simulink model "Quadcopter_Plant_x"  (R2022b)
settings: Solver=FixedStepAuto  StartTime=0.0  StopTime=60  FixedStep=.01  RelTol=1e-3
undefined symbols (not defined in the file): CdProp, Cdx, Cdy, Cdz, Ct, DiscIntNeverNeededParam, Earth, Ixx, Iyy, Izz, Jr, larm, mass, WGS84
libraries: sharedtransform x2, aerolibtransform2 x1
settings Model: Creator=aaron  LastModifiedBy=aaron
settings DataIOCC: SaveOutput=off  SaveTime=off
settings DebuggingCC: ModelReferenceExtraNoncontSigs=none

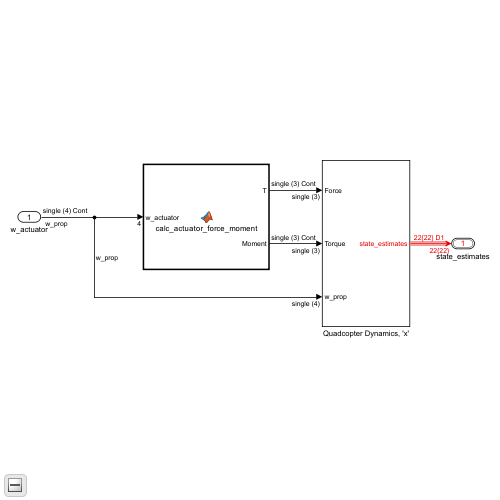
[thumbnail: Simulink's stored preview of the top-level diagram]
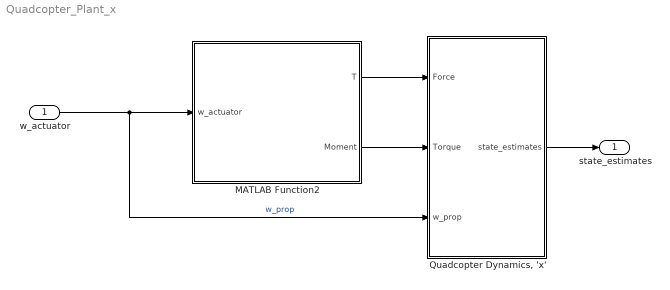
== system Quadcopter_Plant_x ==
  w_actuator : Inport  OutDataTypeStr=single  PortDimensions=4  SampleTime=[0.01,0]
  MATLAB Function2 : MATLAB Function  TreatAsAtomicUnit=on
  "Quadcopter Dynamics, 'x'" : Subsystem
  state_estimates : Outport  OutDataTypeStr=Bus: state_estimates  LockScale=on
  wires:
  MATLAB Function2/1(T) -> "Quadcopter Dynamics, 'x'"/1(Force)
  MATLAB Function2/2(Moment) -> "Quadcopter Dynamics, 'x'"/2(Torque)
  w_actuator/1 -> "Quadcopter Dynamics, 'x'"/3(w_prop), MATLAB Function2/1(w_actuator)  "w_prop"
  "Quadcopter Dynamics, 'x'"/1(state_estimates) -> state_estimates/1

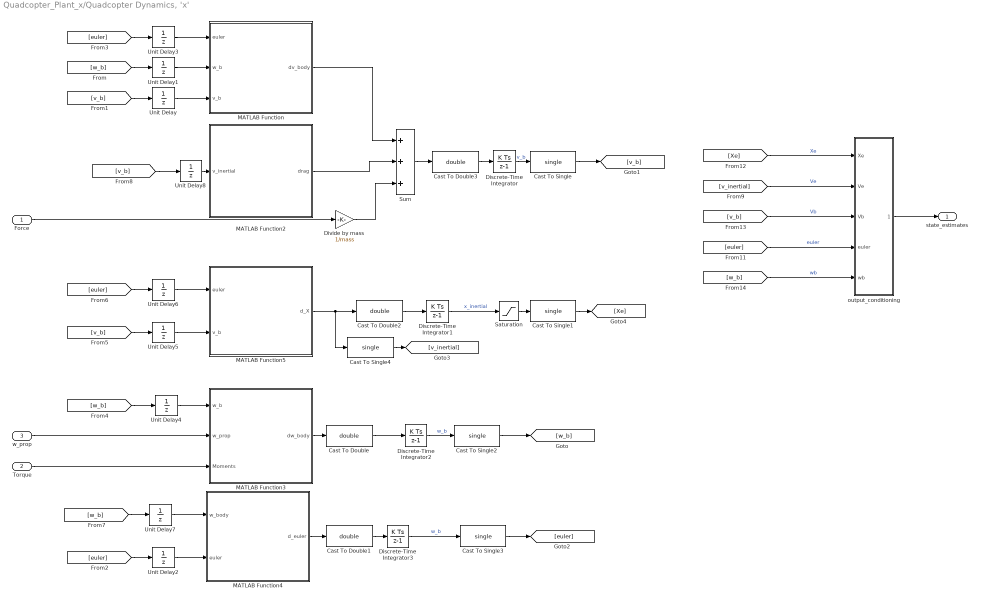
== system Quadcopter_Plant_x/Quadcopter Dynamics, 'x' ==
  Force : Inport  OutDataTypeStr=single
  Torque : Inport  Port=2  OutDataTypeStr=single
  w_prop : Inport  Port=3  OutDataTypeStr=single
  Cast To Double{,1..3} (4 alike) : DataTypeConversion  OutDataTypeStr=double  SaturateOnIntegerOverflow=off  RndMeth=Floor
  Cast To Single{,1..4} (5 alike) : DataTypeConversion  OutDataTypeStr=single  SaturateOnIntegerOverflow=off  RndMeth=Floor
  Discrete-Time Integrator : DiscreteIntegrator  SampleTime=.01  OutDataTypeStr=single  ICPrevOutput=DiscIntNeverNeededParam  ICPrevScaledInput=DiscIntNeverNeededParam
  Discrete-Time Integrator1 : DiscreteIntegrator  SampleTime=.01  OutDataTypeStr=single  LimitOutput=on  UpperSaturationLimit=[inf inf 0]  LowerSaturationLimit=[-inf -inf -inf]  ICPrevOutput=DiscIntNeverNeededParam  ICPrevScaledInput=DiscIntNeverNeededParam
  Discrete-Time Integrator2 : DiscreteIntegrator  SampleTime=.01  OutDataTypeStr=single  ICPrevOutput=DiscIntNeverNeededParam  ICPrevScaledInput=DiscIntNeverNeededParam
  Discrete-Time Integrator3 : DiscreteIntegrator  SampleTime=.01  OutDataTypeStr=single  ICPrevOutput=DiscIntNeverNeededParam  ICPrevScaledInput=DiscIntNeverNeededParam
  Divide by mass : Gain  Gain=1/mass  OutDataTypeStr=single
  MATLAB Function : MATLAB Function  TreatAsAtomicUnit=on
  MATLAB Function2 : MATLAB Function  TreatAsAtomicUnit=on
  MATLAB Function3 : MATLAB Function  TreatAsAtomicUnit=on
  MATLAB Function4 : MATLAB Function  TreatAsAtomicUnit=on
  MATLAB Function5 : MATLAB Function  TreatAsAtomicUnit=on
  Saturation : Saturate  UpperLimit=[inf inf 0]  LowerLimit=-inf
  Sum : Sum  Inputs=+++
  Unit Delay{,1..8} (9 alike) : UnitDelay  SampleTime=-1  HasFrameUpgradeWarning=on
  output_conditioning : Subsystem
  state_estimates : Outport  OutDataTypeStr=Bus: state_estimates  LockScale=on
  wires:
  Divide by mass/1 -> Sum/3
  Torque/1 -> MATLAB Function3/3(Moments)
  MATLAB Function3/1(dw_body) -> Cast To Double/1
  Discrete-Time Integrator1/1 -> Saturation/1  "x_inertial"
  [v_b] -> Unit Delay8/1
  Unit Delay8/1 -> MATLAB Function2/1(v_inertial)
  MATLAB Function5/1(d_X) -> Cast To Single4/1, Cast To Double2/1
  Unit Delay7/1 -> MATLAB Function4/1(w_body)
  [w_b] -> Unit Delay7/1
  Unit Delay6/1 -> MATLAB Function5/1(euler)
  [euler] -> Unit Delay6/1
  Unit Delay5/1 -> MATLAB Function5/2(v_b)
  [v_b] -> Unit Delay5/1
  Unit Delay4/1 -> MATLAB Function3/1(w_b)
  [w_b] -> Unit Delay4/1
  w_prop/1 -> MATLAB Function3/2(w_prop)
  [euler] -> Unit Delay2/1
  Unit Delay3/1 -> MATLAB Function/1(euler)
  [euler] -> Unit Delay3/1
  Unit Delay2/1 -> MATLAB Function4/2(euler)
  MATLAB Function4/1(d_euler) -> Cast To Double1/1
  [v_b] -> Unit Delay/1
  Discrete-Time Integrator/1 -> Cast To Single/1  "v_b"
  [w_b] -> Unit Delay1/1
  Unit Delay1/1 -> MATLAB Function/2(w_b)
  Discrete-Time Integrator2/1 -> Cast To Single2/1  "w_b"
  Sum/1 -> Cast To Double3/1
  Force/1 -> Divide by mass/1
  Unit Delay/1 -> MATLAB Function/3(v_b)
  MATLAB Function2/1(drag) -> Sum/2
  MATLAB Function/1(dv_body) -> Sum/1
  Saturation/1 -> Cast To Single1/1
  [Xe] -> output_conditioning/1(Xe)  "Xe"
  [v_inertial] -> output_conditioning/2(Ve)  "Ve"
  [v_b] -> output_conditioning/3(Vb)  "Vb"
  [euler] -> output_conditioning/4(euler)  "euler"
  [w_b] -> output_conditioning/5(wb)  "wb"
  output_conditioning/1(state_estimates) -> state_estimates/1
  Cast To Single/1 -> [v_b]
  Cast To Single1/1 -> [Xe]
  Cast To Single2/1 -> [w_b]
  Discrete-Time Integrator3/1 -> Cast To Single3/1  "w_b"
  Cast To Single3/1 -> [euler]
  Cast To Double/1 -> Discrete-Time Integrator2/1
  Cast To Double1/1 -> Discrete-Time Integrator3/1
  Cast To Single4/1 -> [v_inertial]
  Cast To Double2/1 -> Discrete-Time Integrator1/1
  Cast To Double3/1 -> Discrete-Time Integrator/1

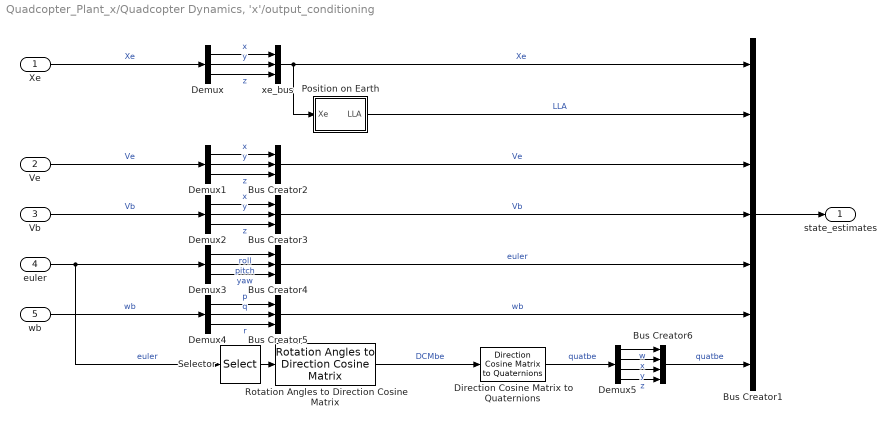
== system Quadcopter_Plant_x/Quadcopter Dynamics, 'x'/output_conditioning ==
  Xe : Inport
  Ve : Inport  Port=2
  Vb : Inport  Port=3
  euler : Inport  Port=4
  wb : Inport  Port=5
  Bus Creator1 : BusCreator  Inputs=7  OutDataTypeStr=Bus: state_estimates
  Bus Creator2 : BusCreator  Inputs=3  OutDataTypeStr=Bus: Velocity
  Bus Creator3 : BusCreator  Inputs=3  OutDataTypeStr=Bus: Velocity
  Bus Creator4 : BusCreator  Inputs=3  OutDataTypeStr=Bus: euler
  Bus Creator5 : BusCreator  Inputs=3  OutDataTypeStr=Bus: body_rates
  Bus Creator6 : BusCreator  Inputs=4  OutDataTypeStr=Bus: quat
  Demux{,1..4} (5 alike) : Demux  Outputs=3
  Demux5 : Demux
  Direction Cosine Matrix to Quaternions : sharedtransform/Direction Cosine Matrix  to Quaternions  aMode=0  action=None  tolerance=eps(2)
      settings: LibrarySourceBlock=|
      | aerolibtransform2/Direction Cosine Matrix
      | to Quaternions
  Position on Earth : Subsystem  Priority=1  TreatAsAtomicUnit=on
  Rotation Angles to Direction Cosine Matrix : sharedtransform/Rotation Angles to Direction Cosine Matrix  rotationOrder=ZYX  aMode=aMode
  Selector : Selector  InputPortWidth=3  IndexOptions=Index vector (dialog)  Indices=[3 2 1]  OutputSizes=1
  xe_bus : BusCreator  Inputs=3  OutDataTypeStr=Bus: Position
  state_estimates : Outport  OutDataTypeStr=Bus: state_estimates  LockScale=on
  wires:
  euler/1 -> Demux3/1, Selector/1  "euler"
  Bus Creator1/1 -> state_estimates/1
  Position on Earth/1(LLA) -> Bus Creator1/2  "LLA"
  Selector/1 -> Rotation Angles to Direction Cosine Matrix/1
  Xe/1 -> Demux/1  "Xe"
  Demux/1 -> xe_bus/1  "x"
  Demux/2 -> xe_bus/2  "y"
  Demux/3 -> xe_bus/3  "z"
  xe_bus/1 -> Bus Creator1/1, Position on Earth/1(Xe)  "Xe"
  Demux1/1 -> Bus Creator2/1  "x"
  Demux1/2 -> Bus Creator2/2  "y"
  Demux1/3 -> Bus Creator2/3  "z"
  Ve/1 -> Demux1/1  "Ve"
  Bus Creator2/1 -> Bus Creator1/3  "Ve"
  Demux2/3 -> Bus Creator3/3  "z"
  Demux2/2 -> Bus Creator3/2  "y"
  Demux2/1 -> Bus Creator3/1  "x"
  Bus Creator3/1 -> Bus Creator1/4  "Vb"
  Vb/1 -> Demux2/1  "Vb"
  Demux3/1 -> Bus Creator4/1  "roll"
  Demux3/2 -> Bus Creator4/2  "pitch"
  Demux3/3 -> Bus Creator4/3  "yaw"
  Bus Creator4/1 -> Bus Creator1/5  "euler"
  wb/1 -> Demux4/1  "wb"
  Bus Creator5/1 -> Bus Creator1/6  "wb"
  Demux4/1 -> Bus Creator5/1  "p"
  Demux4/2 -> Bus Creator5/2  "q"
  Demux4/3 -> Bus Creator5/3  "r"
  Rotation Angles to Direction Cosine Matrix/1 -> Direction Cosine Matrix to Quaternions/1  "DCMbe"
  Demux5/1 -> Bus Creator6/1  "w"
  Demux5/2 -> Bus Creator6/2  "x"
  Demux5/3 -> Bus Creator6/3  "y"
  Demux5/4 -> Bus Creator6/4  "z"
  Bus Creator6/1 -> Bus Creator1/7  "quatbe"
  Direction Cosine Matrix to Quaternions/1 -> Demux5/1  "quatbe"

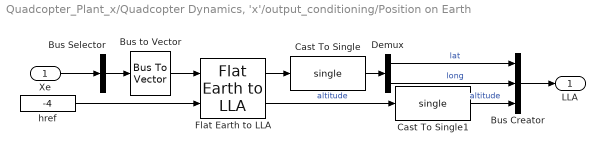
== system Quadcopter_Plant_x/Quadcopter Dynamics, 'x'/output_conditioning/Position on Earth ==
  Xe : Inport  OutDataTypeStr=Bus: Position  Unit=m
  Bus Creator : BusCreator  Inputs=3  OutDataTypeStr=Bus: LLA
  Bus Selector : BusSelector  OutputSignals=x,y,z  OutputAsBus=on
  Bus to Vector : BusToVector
  Cast To Single : DataTypeConversion  OutDataTypeStr=single  SaturateOnIntegerOverflow=off  RndMeth=Floor
  Cast To Single1 : DataTypeConversion  OutDataTypeStr=single  SaturateOnIntegerOverflow=off  RndMeth=Floor
  Demux : Demux  Outputs=2
  Flat Earth to LLA : aerolibtransform2/Flat Earth to LLA  units=Metric (MKS)  ptype=Earth (WGS84)  F=1/298.257223563  R=6378137  refPosPort=off  LL0=[-122.389977, 37.615223]  psi=0
  href : Constant  Value=-4
  LLA : Outport  OutDataTypeStr=Bus: LLA  VectorParamsAs1DForOutWhenUnconnected=off
  wires:
  Bus Creator/1 -> LLA/1
  href/1 -> Flat Earth to LLA/2
  Demux/2 -> Bus Creator/2  "long"
  Flat Earth to LLA/1 -> Cast To Single/1
  Demux/1 -> Bus Creator/1  "lat"
  Flat Earth to LLA/2 -> Cast To Single1/1  "altitude"
  Xe/1 -> Bus Selector/1
  Bus Selector/1 -> Bus to Vector/1
  Bus to Vector/1 -> Flat Earth to LLA/1
  Cast To Single/1 -> Demux/1
  Cast To Single1/1 -> Bus Creator/3  "altitude"

== matlab function Quadcopter_Plant_x/MATLAB Function2 ==
  data: w_actuator input single; T output single size=3; Moment output single size=3; Ct parameter single; larm parameter single; CdProp parameter single
function [T, Moment] = calc_actuator_force_moment(w_actuator, Ct, larm, CdProp)

K = Ct;
L_arm = larm;
C = CdProp;


w1 = w_actuator(1)^2;
w2 = w_actuator(2)^2;
w3 = w_actuator(3)^2;
w4 = w_actuator(4)^2;

T = [0; 0; -K * (sum(w_actuator.^2))];
L = K*L_arm*(-w1 + w2 + w3 - w4);
M = K*L_arm*(-w1 - w2 + w3 + w4);
N = C*(-w1 - w3 + w2 + w4);

Moment = [L; M; N];

== matlab function Quadcopter_Plant_x/Quadcopter Dynamics, 'x'/MATLAB Function ==
  data: euler input; dv_body output size=3; w_b input; v_b input; g parameter
function dv_body = calc_body_vel_change(euler, w_b, v_b, g)

u = v_b(1);
v = v_b(2);
w = v_b(3);

theta = euler(2);
phi = euler(1);
psi = euler(3);

p = w_b(1);
q = w_b(2);
r = w_b(3);


du = -g*sin(theta)+r*v - q*w;
dv = g*sin(phi)*cos(theta) - r*u + p*w;
dw = g*cos(phi)*cos(theta) + q*u - p*v;

dv_body = [du; dv; dw];

== matlab function Quadcopter_Plant_x/Quadcopter Dynamics, 'x'/MATLAB Function2 ==
  data: v_inertial input single; drag output single size=3; Cdx parameter single; Cdy parameter single; Cdz parameter single; mass parameter single
function drag = calc_drag(v_inertial, Cdx, Cdy, Cdz, mass)

dx = v_inertial(1);
dy = v_inertial(2);
dz = v_inertial(3);

Fd_x = -(1/mass)*Cdx*dx;
Fd_y = -(1/mass)*Cdy*dy;
Fd_z = -(1/mass)*Cdz*dz;

drag = [Fd_x; Fd_y; Fd_z];

== matlab function Quadcopter_Plant_x/Quadcopter Dynamics, 'x'/MATLAB Function3 ==
  data: w_b input single; dw_body output single size=3; w_prop input single; Moments input single; Ixx parameter single; Iyy parameter single; Izz parameter single; Jr parameter single
function dw_body = calc_body_rate_change(w_b, w_prop, Moments, ...
Ixx, Iyy, Izz, Jr)

L = Moments(1);
M = Moments(2);
N = Moments(3);

omega_p = -w_prop(1) + w_prop(2) - w_prop(3) + w_prop(4);


p = w_b(1);
q = w_b(2);
r = w_b(3);

dp = (1/Ixx)*(L + (Iyy - Izz)*q*r) + q*omega_p*Jr/Ixx;
dq = (1/Iyy)*(M + (Izz - Ixx)*p*r) - p*omega_p*Jr/Iyy;
% dp = (1/Ixx)*(L + (Iyy - Izz)*q*r);
% dq = (1/Iyy)*(M + (Izz - Ixx)*p*r);
dr = (1/Izz)*(N + (Ixx - Iyy)*p*q);

dw_body = single([dp; dq; dr]);

== matlab function Quadcopter_Plant_x/Quadcopter Dynamics, 'x'/MATLAB Function4 ==
  data: w_body input single; d_euler output single size=3; euler input single
function d_euler = calc_euler_change(w_body, euler)

phi = euler(1);
theta = euler(2);
psi = euler(3);

p = w_body(1);
q = w_body(2);
r = w_body(3);

d_phi = p + (q*sin(phi) + r*cos(phi)) * tan(theta);
d_theta = q*cos(phi) - r*sin(phi);
d_psi = (q*sin(phi) + r*cos(phi))*(1/cos(theta));

d_euler = [d_phi; d_theta; d_psi];

== matlab function Quadcopter_Plant_x/Quadcopter Dynamics, 'x'/MATLAB Function5 ==
  data: euler input single; d_X output single size=3; v_b input single
function d_X = calc_inertial_velocity(euler, v_b)

phi = euler(1);
theta = euler(2);
psi = euler(3);

u = v_b(1);
v = v_b(2);
w = v_b(3);

dx = cos(theta)*cos(psi)*u + (-cos(phi)*sin(psi) + sin(phi)*sin(theta)*cos(psi))*v +...
    (sin(phi)*sin(psi)+cos(phi)*sin(theta)*cos(psi))*w;

dy = cos(theta)*sin(psi)*u + (cos(phi)*cos(psi)+sin(phi)*sin(theta)*sin(psi))*v + ...
    (-sin(phi)*cos(psi)+cos(phi)*sin(theta)*sin(psi))*w;

dz = (-sin(theta)*u+sin(phi)*cos(theta)*v+cos(phi)*cos(theta)*w);
d_X = [dx; dy; dz];
